simulink model "exampleSpecificVolume"  (Simulink 7.6)
settings: Solver=ode45  StartTime=0.0  StopTime=10.0  RelTol=1e-3
libraries: carnot x4
settings Model: Creator=drhf  LastModifiedBy=drhf

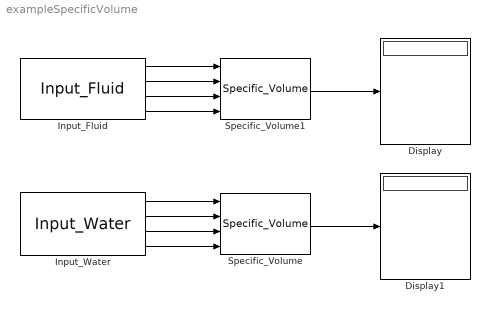
== system exampleSpecificVolume ==
  Display : Display
  Display1 : Display
  Input_Fluid : carnot/Basic/Material_Properties/Input_Fluid  SystemSampleTime=-1  fluid=water  T=[10:10:50]  p=1e5  x=0.005
  Input_Water : carnot/Basic/Material_Properties/Input_Water  SystemSampleTime=-1  T=10:20:90  p=2e6  xd=0
  Specific_Volume : carnot/Basic/Material_Properties/Specific_Volume  SystemSampleTime=-1
  Specific_Volume1 : carnot/Basic/Material_Properties/Specific_Volume  SystemSampleTime=-1
  wires:
  Input_Fluid/1 -> Specific_Volume1/1
  Input_Fluid/2 -> Specific_Volume1/2
  Input_Fluid/3 -> Specific_Volume1/3
  Input_Fluid/4 -> Specific_Volume1/4
  Specific_Volume1/1 -> Display/1
  Input_Water/1 -> Specific_Volume/1
  Input_Water/2 -> Specific_Volume/2
  Input_Water/3 -> Specific_Volume/3
  Input_Water/4 -> Specific_Volume/4
  Specific_Volume/1 -> Display1/1
